simulink model "bioreactor_openloop"  (R2019b)
settings: Solver=VariableStepAuto  StartTime=0.0  StopTime=10.0  MaxStep=1e-3  RelTol=1e-3
values from neighbouring files (symbols this model uses):
  A = 0.0056    [bioreactor_EOM.m]
  C = 2.6e-8    (= 2.6e-08)    [bioreactor_EOM.m]
  R = 2.9e7    (= 29000000)    [bioreactor_EOM.m]
  r = 0.012    [bioreactor_EOM.m]
settings Model: Creator=lutkus  LastModifiedBy=lutkus

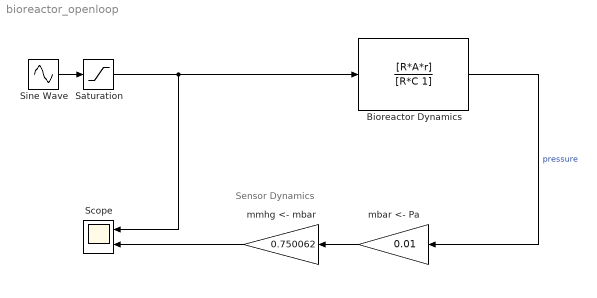
== system bioreactor_openloop ==
  note: Sensor Dynamics
  "Bioreactor Dynamics " : TransferFcn  Numerator=[R*A*r]  Denominator=[R*C 1]
  Saturation : Saturate  UpperLimit=1  LowerLimit=0
  Scope : Scope  NumInputPorts=2
  Sine Wave : Sin  Frequency=2*pi  SampleTime=0
  mbar <- Pa : Gain  Gain=0.01
  mmhg <- mbar : Gain  Gain=0.750062
  wires:
  mbar <- Pa/1 -> mmhg <- mbar/1
  "Bioreactor Dynamics "/1 -> mbar <- Pa/1  "pressure"
  mmhg <- mbar/1 -> Scope/2
  Sine Wave/1 -> Saturation/1
  Saturation/1 -> Scope/1, "Bioreactor Dynamics "/1
